simulink model "Model_4"  (R2020b)
settings: Solver=VariableStepAuto  StartTime=0.0  StopTime=10.0  RelTol=1e-3
settings Model: Creator=Akarsh  LastModifiedBy=Akarsh

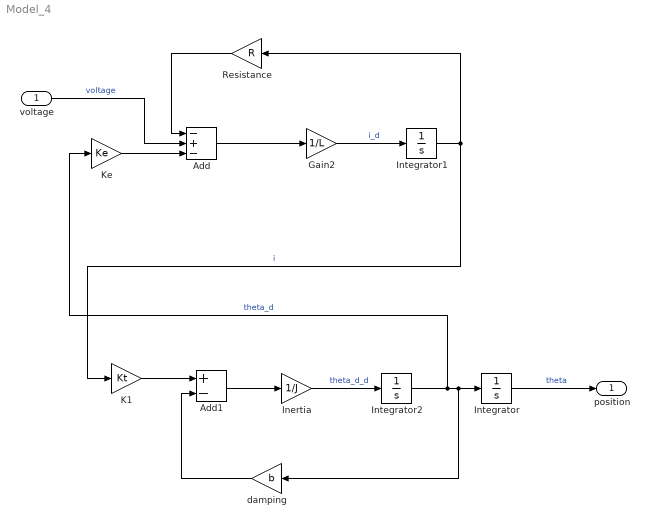
== system Model_4 ==
  voltage : Inport
  Add : Sum  Inputs=-+-
  Add1 : Sum  Inputs=+-
  Gain2 : Gain  Gain=1/L  mask{L=2.75*10^-6}
  Inertia : Gain  Gain=1/J  mask{J=3.22*10^-6}
  Integrator : Integrator
  Integrator1 : Integrator
  Integrator2 : Integrator
  K1 : Gain  Gain=Kt  mask{Kt=0.0274}
  Ke : Gain  Gain=Ke  mask{Ke=0.0274}
  Resistance : Gain  Gain=R  mask{R=4}
  damping : Gain  Gain=b  mask{b=3.5*10^-6}
  position : Outport
  wires:
  K1/1 -> Add1/1
  damping/1 -> Add1/2
  Add1/1 -> Inertia/1
  Inertia/1 -> Integrator2/1  "theta_d_d"
  Integrator2/1 -> Ke/1, damping/1, Integrator/1  "theta_d"
  Integrator/1 -> position/1  "theta"
  Ke/1 -> Add/3
  Add/1 -> Gain2/1
  Gain2/1 -> Integrator1/1  "i_d"
  Integrator1/1 -> Resistance/1, K1/1  "i"
  Resistance/1 -> Add/1
  voltage/1 -> Add/2  "voltage"
